simulink model "ModificadoSimulacionControlSysNoLineal_Simplificado_Qube2"  (R2018b)
settings: Solver=ode3  StartTime=0.0  StopTime=10  FixedStep=0.001  RelTol=1e-3  EnableMultiTasking=on
values from neighbouring files (symbols this model uses):
  betaP = 0.0005    [ParametrosModeloNOlinealPendulo.m]
  betaR = 0.0015    [ParametrosModeloNOlinealPendulo.m]
  g = 9.8    [ParametrosModeloNOlinealPendulo.m]
  Jb = Mb*Lb^2/12    (= 5.71979166667e-05)    [ParametrosModeloNOlinealPendulo.m]
  Jp = Mp*(Lcm*2)^2/12    (= 3.3282e-05)    [ParametrosModeloNOlinealPendulo.m]
  K = Keq*inv(P)    [ParametrosModeloNOlinealPendulo.m]
  kc = dcgain(salBra)    [ParametrosModeloNOlinealPendulo.m]
  km = 0.042    [ParametrosModeloNOlinealPendulo.m]
  Lb = 0.085    [ParametrosModeloNOlinealPendulo.m]
  Lcm = 0.129/2    (= 0.0645)    [ParametrosModeloNOlinealPendulo.m]
  Mp = 0.024    [ParametrosModeloNOlinealPendulo.m]
  Rm = 8.4    [ParametrosModeloNOlinealPendulo.m]
libraries: simulink x4, simulink_extras x3, vrlib x1
settings Model: Creator=Alejandra  LastModifiedBy=AlfredoMaussa
settings DataIOCC: LimitDataPoints=on  SaveFormat=Array
settings OptimizationCC: LifeSpan=inf
settings DebuggingCC: SFUnexpectedBacktrackingDiag=warning  SFNoUnconditionalDefaultTransitionDiag=warning  SFExecutionAtInitializationDiag=none
settings HardwareCC: ProdBitPerPointer=32  ProdBitPerSizeT=32  ProdBitPerPtrDiffT=32  ProdLargestAtomicFloat=None  ProdIntDivRoundTo=Undefined  ProdEndianess=Unspecified  ProdWordSize=32  ProdHWDeviceType=32-bit Generic
settings ModelReferenceCC: PropagateSignalLabelsOutOfModel=off
settings SFSimCC: SimUseLocalCustomCode=off
settings RTWCC: RTWUseLocalCustomCode=off
settings CodeAppCC: StateflowObjectComments=on
settings GRTTargetCC: TargetLangStandard=C89/C90 (ANSI)  GeneratePreprocessorConditionals=Disable all
settings ConfigComp: CovMetricSettings=dw  CovHtmlReporting=on  CovSaveCumulativeToWorkspaceVar=on  CovSaveSingleToWorkspaceVar=on  CovExternalEMLEnable=off

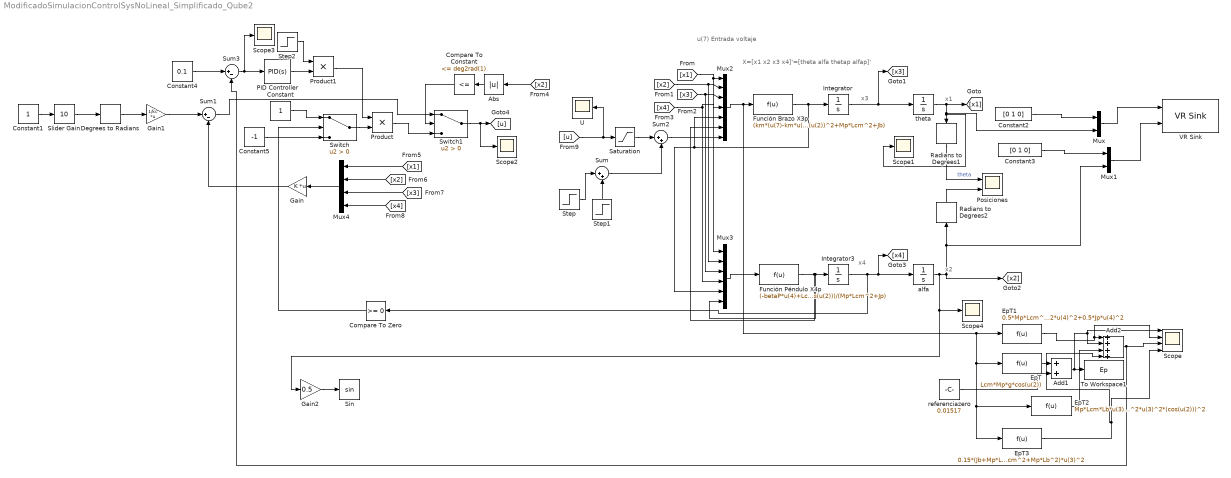
== system ModificadoSimulacionControlSysNoLineal_Simplificado_Qube2 ==
  note: u(7) Entrada voltaje
  note: x4
  note: x3
  note: x2
  note: x1
  note: X=[x1 x2 x3 x4]'=[theta alfa thetap alfap]'
  Abs : Abs
  Add1 : Sum
  Add2 : Sum  Inputs=++++
  Compare To Constant : simulink/Logic and Bit Operations/Compare To Constant  relop=<=  const=deg2rad(1)  OutDataTypeStr=boolean
  Compare To Zero : simulink/Logic and Bit Operations/Compare To Zero  relop=>=  OutDataTypeStr=boolean
  Constant : Constant
  Constant1 : Constant
  Constant2 : Constant  Value=[0 1 0]
  Constant3 : Constant  Value=[0 1 0]
  Constant4 : Constant  Value=0.1
  Constant5 : Constant  Value=-1
  Degrees to Radians : simulink_extras/Transformations/Degrees to Radians
  EpT : Fcn  Expr=Lcm*Mp*g*cos(u(2))
  EpT1 : Fcn  Expr=0.5*Mp*Lcm^2*u(4)^2+0.5*Jp*u(4)^2
  EpT2 : Fcn  Expr=Mp*Lcm*Lb*u(3)*u(4)*cos(u(2))+0.5*Mp*Lcm^2*u(3)^2*(cos(u(2)))^2
  EpT3 : Fcn  Expr=0.15*(Jb+Mp*Lcm^2+Mp*Lb^2)*u(3)^2
  Función Brazo X3p : Fcn  Expr=(km*(u(7)-km*u(3))/(Rm)-betaR*u(3)+(Lb*Lcm*Mp*u(4)^2*sin(u(2)))-Lb*Lcm*Mp*u(6)*cos(u(2))-2*Lcm^2*Mp*u(3)*u(4)*cos(u(2))*sin(u(2)))/(Mp*Lb^2-Mp*Lcm^2*cos(u(2))^2+Mp*Lcm^2+Jb)
  Función Péndulo X4p : Fcn  Expr=(-betaP*u(4)+Lcm^2*Mp*Lcm^2*cos(u(2))*sin(u(2))+Lcm*Mp*g*sin(u(2))-Lb*Lcm*Mp*u(5)*cos(u(2)))/(Mp*Lcm^2+Jp)
  Gain : Gain  Gain=K  Multiplication=Matrix(K*u)
  Gain1 : Gain  Gain=1/kc  Multiplication=Matrix(K*u)
  Gain2 : Gain  Gain=0.5
  Integrator : Integrator
  Integrator3 : Integrator
  Mux : Mux  Inputs=2
  Mux1 : Mux  Inputs=2
  Mux2 : Mux  Inputs=7
  Mux3 : Mux  Inputs=6
  Mux4 : Mux
  PID Controller : simulink/Continuous/PID Controller  Controller=PID  Form=Parallel  TimeDomain=Continuous-time  SampleTime=-1  IntegratorMethod=Forward Euler  FilterMethod=Forward Euler  ControllerParametersSource=internal  P=100  I=100  D=0  UseFilter=on  N=100  TunerSelectOption=Transfer Function Based (PID Tuner App)  InitialConditionSource=internal  InitialConditionForIntegrator=0  InitialConditionForFilter=0  DifferentiatorICPrevScaledInput=0  ExternalReset=none  TrackingMode=off  Kt=1  LimitOutput=off  UpperSaturationLimit=inf  LowerSaturationLimit=-inf  LinearizeAsGain=on  AntiWindupMode=none  Kb=1  POutMin=[]  POutMax=[]  IOutMin=[]  IOutMax=[]  DOutMin=[]  DOutMax=[]  NOutMin=[]  NOutMax=[]  SumOutMin=[]  SumOutMax=[]  SaturationOutMin=[]  SaturationOutMax=[]  PParamMin=[]  PParamMax=[]  IParamMin=[]  IParamMax=[]  DParamMin=[]  DParamMax=[]  NParamMin=[]  NParamMax=[]  KbParamMin=[]  KbParamMax=[]  KtParamMin=[]  KtParamMax=[]  KbOutMin=[]  KbOutMax=[]  KtOutMin=[]  KtOutMax=[]  IntegratorOutMin=[]  IntegratorOutMax=[]  FilterOutMin=[]  FilterOutMax=[]  SumI1OutMin=[]  SumI1OutMax=[]  SumI2OutMin=[]  SumI2OutMax=[]  SumI3OutMin=[]  SumI3OutMax=[]  SumI4OutMin=[]  SumI4OutMax=[]  SumDOutMin=[]  SumDOutMax=[]  DifferentiatorOutMin=[]  DifferentiatorOutMax=[]  FilterDiffOutCoefMin=[]  FilterDiffOutCoefMax=[]  ReciprocalOutMin=[]  ReciprocalOutMax=[]  SumDenOutMin=[]  SumDenOutMax=[]  SumNumOutMin=[]  SumNumOutMax=[]  DivideOutMin=[]  DivideOutMax=[]  IntegratorContinuousStateAttributes=''  IntegratorStateMustResolveToSignalObject=off  IntegratorRTWStateStorageClass=Auto  FilterContinuousStateAttributes=''  FilterStateMustResolveToSignalObject=off  FilterRTWStateStorageClass=Auto  ParallelPVariant=InternalParameters  IdealPVariant=Disabled  IVariant=InternalParameters  DVariant=InternalParameters  IntegratorVariant=Continuous  SatVariant=Disabled  AWVariant=Passthrough  PCopyVariant=Disabled  TRVariant=Disabled  FdbkBlocksVariant=Forward  IdealPFdbkVariant=Disabled  SatFdbkVariant=Disabled  DerivativeFilterVariant=ContFilter  NVariant=InternalParameters  NCopyVariant=Disabled  FilterICVariant=InternalICsFilter  IntegratorICVariant=InternalICs  ExternalResetVariant=Disabled  TRSumVariant=Passthrough  SumFdbkVariant=Disabled  SumVariant=Sum_PID
  Posiciones : Scope  NumInputPorts=2
  Product : Product
  Product1 : Product
  Radians to Degrees1 : simulink_extras/Transformations/Radians to Degrees
  Radians to Degrees2 : simulink_extras/Transformations/Radians to Degrees
  Saturation : Saturate  UpperLimit=100  LowerLimit=-100
  Scope : Scope  NumInputPorts=4
  Scope{1..4} (4 alike) : Scope
  Sin : Trigonometry
  Slider Gain : simulink/Math Operations/Slider Gain  gain=10  low=-90  high=90
  Step : Step  Time=0.01  After=0.01  SampleTime=0
  Step1 : Step  Time=0  After=-0.01  SampleTime=0
  Step2 : Step  SampleTime=0
  Sum : Sum  Inputs=|++
  Sum1 : Sum  Inputs=|+-
  Sum2 : Sum  Inputs=|++
  Sum3 : Sum  Inputs=|+-
  Switch : Switch  Criteria=u2 > Threshold
  Switch1 : Switch  Criteria=u2 > Threshold
  To Workspace1 : ToWorkspace  VariableName=Ep  SaveFormat=Timeseries  SampleTime=-1
  U : Scope
  VR Sink : vrlib/VR Sink  InstantiateOnLoad=on  SampleTime=-1  ViewEnable=on  RemoteChange=off  RemoteView=off  FieldsWritten=Phi.rotation.4.1.1.double#Theta.rotation.4.1.1.double  WorldFileName=FurutaAnimacion.WRL  AutoView=off  VideoDimensions=[]  AllowVariableSize=off
      settings: SourceProductBaseCode=VR
  alfa : Integrator
  referenciazero : Constant  Value=0.01517
  theta : Integrator
  wires:
  Integrator/1 -> [x3], theta/1
  Función Brazo X3p/1 -> Mux3/5, Mux2/5, Integrator/1
  Mux2/1 -> EpT3/1, EpT2/1, EpT/1, EpT1/1, Función Brazo X3p/1
  Función Péndulo X4p/1 -> Mux3/6, Integrator3/1, Mux2/6
  theta/1 -> Mux/2, Scope1/1, Radians to Degrees1/1, [x1]
  [x1] -> Mux3/1, Mux2/1
  [x2] -> Mux3/2, Mux2/2
  [x3] -> Mux3/3, Mux2/3
  [x4] -> Mux2/4, Mux3/4
  Mux3/1 -> Función Péndulo X4p/1
  Slider Gain/1 -> Degrees to Radians/1
  Constant1/1 -> Slider Gain/1
  Degrees to Radians/1 -> Gain1/1
  Abs/1 -> Compare To Constant/1
  [x2] -> Abs/1
  [x2] -> Mux4/2
  [x1] -> Mux4/1
  [x3] -> Mux4/3
  [x4] -> Mux4/4
  Mux4/1 -> Gain/1
  [u] -> U/1, Saturation/1
  Step/1 -> Sum/1
  Step1/1 -> Sum/2
  Sum/1 -> Sum2/2
  Sum2/1 -> Mux2/7
  Radians to Degrees2/1 -> Posiciones/2
  Saturation/1 -> Sum2/1
  Constant3/1 -> Mux1/1
  Mux1/1 -> VR Sink/2
  Constant2/1 -> Mux/1
  Mux/1 -> VR Sink/1
  Radians to Degrees1/1 -> Posiciones/1  "theta"
  Sum1/1 -> Switch1/1
  Compare To Zero/1 -> Switch/2
  Switch/1 -> Product/2
  Compare To Constant/1 -> Switch1/2
  Gain1/1 -> Sum1/1
  Gain/1 -> Sum1/2
  Product/1 -> Switch1/3
  Integrator3/1 -> Compare To Zero/1, [x4], alfa/1
  Constant5/1 -> Switch/3
  Constant/1 -> Switch/1
  EpT/1 -> Add1/1
  referenciazero/1 -> Add1/2
  Add1/1 -> Add2/2, Scope/1, To Workspace1/1
  Add2/1 -> Sum3/2, Scope/3
  EpT1/1 -> Add2/1, Scope/2
  EpT2/1 -> Add2/3
  EpT3/1 -> Add2/4, Scope/4
  Switch1/1 -> Scope2/1, [u]
  Gain2/1 -> Sin/1
  alfa/1 -> Gain2/1, Scope4/1, [x2], Mux1/2, Radians to Degrees2/1
  Constant4/1 -> Sum3/1
  Step2/1 -> Product1/1
  Product1/1 -> Product/1
  Sum3/1 -> Scope3/1, PID Controller/1
  PID Controller/1 -> Product1/2
